simulink model "Magman_PID"  (R2016b)
settings: Solver=VariableStepAuto  StartTime=0.0  StopTime=60  RelTol=1e-3
values from neighbouring files (symbols this model uses):
  a = 5.713e-09    [LQI_script.m]    (also in PID_script.m = 4.367e-09; fminsim.m = block.InputPort(3).Data; model_generation.m = 4.367e-09)
  b = 0.000324    [LQI_script.m]    (also in PID_script.m = 0.0002827; fminsim.m = block.InputPort(4).Data; model_generation.m = 0.0002827)
  c = 0.0005    [PID_script.m]
  h = 0.01    [LQI_script.m]    (also in PID_script.m; model_generation.m)
  x1 = 0.02525    [LQI_script.m]    (also in PID_script.m; fminsim.m = block.InputPort(5).Data; model_generation.m)
  x2 = 0.05    [LQI_script.m]    (also in PID_script.m; fminsim.m = block.InputPort(6).Data; model_generation.m)
  x3 = 0.0751    [LQI_script.m]    (also in PID_script.m; fminsim.m = block.InputPort(7).Data; model_generation.m)
  x4 = 0.103    [LQI_script.m]    (also in PID_script.m; fminsim.m = block.InputPort(8).Data; model_generation.m)
undefined symbols (not defined in the file or in its folder): Ad, Bd, Cd, Dd, Humusoft, MF634
libraries: simulink x12, dspsrcs4 x1, sldrtlib x1
settings Model: Creator=Andres  LastModifiedBy=ajurisson

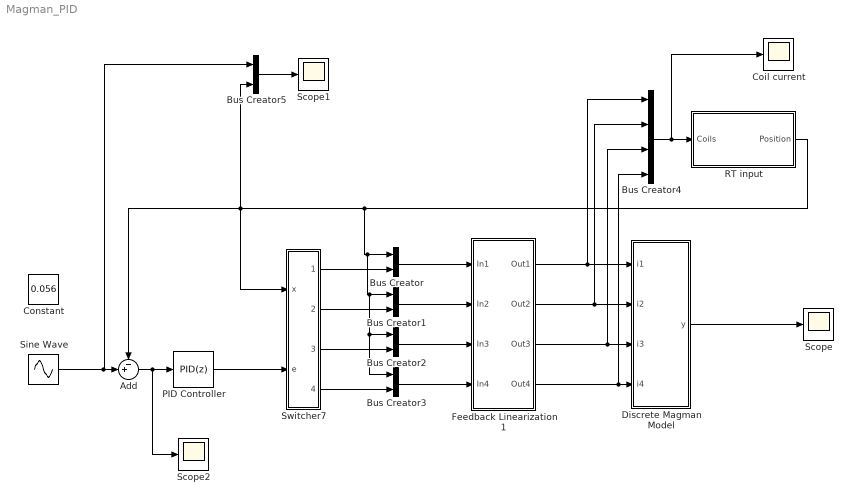
== system Magman_PID ==
  Add : Sum  Inputs=-+|
  Bus Creator{,1..3,5} (5 alike) : BusCreator  Inputs=2
  Bus Creator4 : BusCreator  Inputs=4
  Coil current : Scope
  Constant : Constant  Value=0.056
  Discrete Magman Model : Subsystem
  Feedback Linearization1 : Subsystem
  PID Controller : simulink/Continuous/PID Controller  Controller=PID  TimeDomain=Discrete-time  SampleTime=-1  IntegratorMethod=Trapezoidal  FilterMethod=Trapezoidal  Form=Parallel  UseFilter=on  ControllerParametersSource=internal  P=2.2  I=1  D=5  N=1000  InitialConditionSource=internal  InitialConditionForIntegrator=0  InitialConditionForFilter=0  ExternalReset=none  LimitOutput=off  UpperSaturationLimit=inf  LowerSaturationLimit=-inf  LinearizeAsGain=on  AntiWindupMode=none  Kb=1  TrackingMode=off  Kt=1  PParamMin=[]  PParamMax=[]  IParamMin=[]  IParamMax=[]  DParamMin=[]  DParamMax=[]  NParamMin=[]  NParamMax=[]  KbParamMin=[]  KbParamMax=[]  KtParamMin=[]  KtParamMax=[]  POutMin=[]  POutMax=[]  IOutMin=[]  IOutMax=[]  DOutMin=[]  DOutMax=[]  NOutMin=[]  NOutMax=[]  KbOutMin=[]  KbOutMax=[]  KtOutMin=[]  KtOutMax=[]  IntegratorOutMin=[]  IntegratorOutMax=[]  FilterOutMin=[]  FilterOutMax=[]  SumOutMin=[]  SumOutMax=[]  SumI1OutMin=[]  SumI1OutMax=[]  SumI2OutMin=[]  SumI2OutMax=[]  SumI3OutMin=[]  SumI3OutMax=[]  SumDOutMin=[]  SumDOutMax=[]  SaturationOutMin=[]  SaturationOutMax=[]  IntegratorContinuousStateAttributes=''  IntegratorStateMustResolveToSignalObject=off  IntegratorRTWStateStorageClass=Auto  FilterContinuousStateAttributes=''  FilterStateMustResolveToSignalObject=off  FilterRTWStateStorageClass=Auto  DifferentiatorICPrevScaledInput=0  DifferentiatorOutMin=[]  DifferentiatorOutMax=[]
  RT input : Subsystem  mask{h=0.01, Port=['COM4';'COM5']}
      mask prompts: h "Sample time [s]:"; Port "Serial ports:"
      mask Display: disp('Magman')
  Scope : Scope
  Scope1 : Scope
  Scope2 : Scope
  Sine Wave : Sin  Amplitude=0.032  Bias=0.063  Frequency=1.2  SampleTime=0
  Switcher7 : Subsystem
  wires:
  Add/1 -> Scope2/1, PID Controller/1
  PID Controller/1 -> Switcher7/2(e)
  Switcher7/2(v2) -> Bus Creator1/2
  Switcher7/4(v4) -> Bus Creator3/2
  Switcher7/3(v3) -> Bus Creator2/2
  Switcher7/1(v1) -> Bus Creator/2
  Bus Creator/1 -> Feedback Linearization1/1(In1)
  Bus Creator1/1 -> Feedback Linearization1/2(In2)
  Bus Creator2/1 -> Feedback Linearization1/3(In3)
  Bus Creator3/1 -> Feedback Linearization1/4(In4)
  Feedback Linearization1/1(Out1) -> Bus Creator4/1, Discrete Magman Model/1(i1)
  Feedback Linearization1/3(Out3) -> Bus Creator4/3, Discrete Magman Model/3(i3)
  Feedback Linearization1/4(Out4) -> Bus Creator4/4, Discrete Magman Model/4(i4)
  Bus Creator5/1 -> Scope1/1
  Sine Wave/1 -> Bus Creator5/1, Add/2
  Feedback Linearization1/2(Out2) -> Bus Creator4/2, Discrete Magman Model/2(i2)
  Discrete Magman Model/1(y) -> Scope/1
  Bus Creator4/1 -> Coil current/1, RT input/1(Coils)
  RT input/1(Position) -> Bus Creator3/1, Bus Creator2/1, Bus Creator1/1, Bus Creator/1, Switcher7/1(x), Bus Creator5/2, Add/1

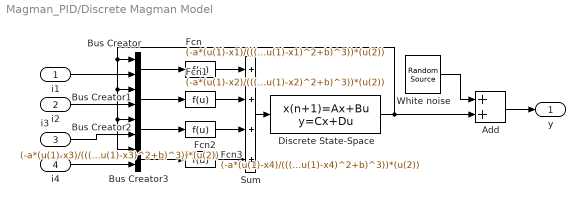
== system Magman_PID/Discrete Magman Model ==
  i1 : Inport
  i2 : Inport  Port=2
  i3 : Inport  Port=3
  i4 : Inport  Port=4
  Add : Sum
  Bus Creator{,1..3} (4 alike) : BusCreator  Inputs=2
  Discrete State-Space : DiscreteStateSpace  A=Ad  B=Bd  C=Cd  D=Dd  SampleTime=h
  Fcn : Fcn  Expr=(-a*(u(1)-x1)/(((u(1)-x1)^2+b)^3))*(u(2))
  Fcn1 : Fcn  Expr=(-a*(u(1)-x2)/(((u(1)-x2)^2+b)^3))*(u(2))
  Fcn2 : Fcn  Expr=(-a*(u(1)-x3)/(((u(1)-x3)^2+b)^3))*(u(2))
  Fcn3 : Fcn  Expr=(-a*(u(1)-x4)/(((u(1)-x4)^2+b)^3))*(u(2))
  Sum : Sum  Inputs=++++
  White noise : dspsrcs4/Random Source  SrcType=Gaussian  NormMethod=Ziggurat  CltLength=12  MinVal=0  MaxVal=1  MeanVal=0  VarVal=pos_var  RepMode=Not repeatable  rawSeed=1  IsInherit=off  SampMode=Discrete  SampTime=h  SampFrame=1  DataType=Double  OutComplex=Real  OutputFrames=off
  y : Outport
  wires:
  Fcn1/1 -> Sum/2
  Add/1 -> y/1
  Bus Creator3/1 -> Fcn3/1
  Bus Creator1/1 -> Fcn1/1
  i1/1 -> Bus Creator/2
  i2/1 -> Bus Creator1/2
  i3/1 -> Bus Creator2/2
  i4/1 -> Bus Creator3/2
  Sum/1 -> Discrete State-Space/1
  Fcn2/1 -> Sum/3
  Bus Creator2/1 -> Fcn2/1
  Fcn/1 -> Sum/1
  Fcn3/1 -> Sum/4
  Bus Creator/1 -> Fcn/1
  Discrete State-Space/1 -> Add/2, Bus Creator3/1, Bus Creator2/1, Bus Creator1/1, Bus Creator/1
  White noise/1 -> Add/1

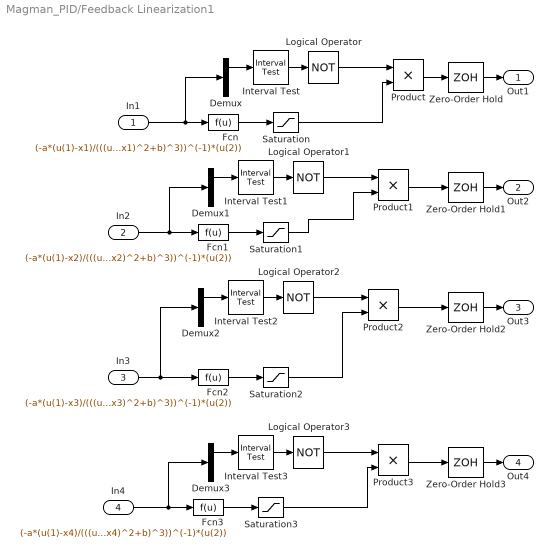
== system Magman_PID/Feedback Linearization1 ==
  In1 : Inport
  In2 : Inport  Port=2
  In3 : Inport  Port=3
  In4 : Inport  Port=4
  Demux{,1..3} (4 alike) : Demux  Outputs=2
  Fcn : Fcn  Expr=(-a*(u(1)-x1)/(((u(1)-x1)^2+b)^3))^(-1)*(u(2))
  Fcn1 : Fcn  Expr=(-a*(u(1)-x2)/(((u(1)-x2)^2+b)^3))^(-1)*(u(2))
  Fcn2 : Fcn  Expr=(-a*(u(1)-x3)/(((u(1)-x3)^2+b)^3))^(-1)*(u(2))
  Fcn3 : Fcn  Expr=(-a*(u(1)-x4)/(((u(1)-x4)^2+b)^3))^(-1)*(u(2))
  Interval Test : simulink/Logic and Bit Operations/Interval Test  IntervalClosedRight=on  uplimit=x1+c  IntervalClosedLeft=on  lowlimit=x1-c  OutDataTypeStr=boolean
  Interval Test1 : simulink/Logic and Bit Operations/Interval Test  IntervalClosedRight=on  uplimit=x2+c  IntervalClosedLeft=on  lowlimit=x2-c  OutDataTypeStr=boolean
  Interval Test2 : simulink/Logic and Bit Operations/Interval Test  IntervalClosedRight=on  uplimit=x3+c  IntervalClosedLeft=on  lowlimit=x3-c  OutDataTypeStr=boolean
  Interval Test3 : simulink/Logic and Bit Operations/Interval Test  IntervalClosedRight=on  uplimit=x4+c  IntervalClosedLeft=on  lowlimit=x4-c  OutDataTypeStr=boolean
  Logical Operator{,1..3} (4 alike) : Logic  Operator=NOT  AllPortsSameDT=off  OutDataTypeStr=boolean
  Product{,1..3} (4 alike) : Product
  Saturation{,1..3} (4 alike) : Saturate  UpperLimit=0.45  LowerLimit=0
  Zero-Order Hold{,1..3} (4 alike) : ZeroOrderHold  SampleTime=-1
  Out1 : Outport
  Out2 : Outport  Port=2
  Out3 : Outport  Port=3
  Out4 : Outport  Port=4
  wires:
  In1/1 -> Demux/1, Fcn/1
  Fcn3/1 -> Saturation3/1
  Fcn2/1 -> Saturation2/1
  Fcn1/1 -> Saturation1/1
  Fcn/1 -> Saturation/1
  Saturation/1 -> Product/2
  Demux/1 -> Interval Test/1
  Interval Test/1 -> Logical Operator/1
  Logical Operator/1 -> Product/1
  Product/1 -> Zero-Order Hold/1
  In2/1 -> Demux1/1, Fcn1/1
  Saturation1/1 -> Product1/2
  Demux1/1 -> Interval Test1/1
  Interval Test1/1 -> Logical Operator1/1
  Logical Operator1/1 -> Product1/1
  Product1/1 -> Zero-Order Hold1/1
  In3/1 -> Demux2/1, Fcn2/1
  Saturation2/1 -> Product2/2
  Demux2/1 -> Interval Test2/1
  Interval Test2/1 -> Logical Operator2/1
  Logical Operator2/1 -> Product2/1
  Product2/1 -> Zero-Order Hold2/1
  In4/1 -> Demux3/1, Fcn3/1
  Saturation3/1 -> Product3/2
  Demux3/1 -> Interval Test3/1
  Interval Test3/1 -> Logical Operator3/1
  Logical Operator3/1 -> Product3/1
  Product3/1 -> Zero-Order Hold3/1
  Zero-Order Hold/1 -> Out1/1
  Zero-Order Hold1/1 -> Out2/1
  Zero-Order Hold2/1 -> Out3/1
  Zero-Order Hold3/1 -> Out4/1

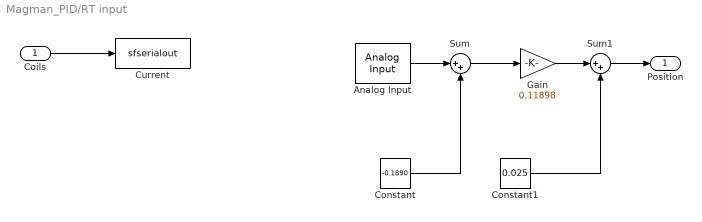
== system Magman_PID/RT input ==
  Coils : Inport
  Analog Input : sldrtlib/Analog Input  SampleTime=h  MaxMissedTicks=100  ShowMissedTicks=off  YieldWhenWaiting=off  DrvName=Humusoft/MF634  DrvAddress=4294967295  DrvOptions=0  Channels=1  RangeMode=2  VoltRange=1  DataType=1
      settings: AttributesFormatString=Humusoft\nMF634 [auto]
  Constant : Constant  Value=-0.1890
  Constant1 : Constant  Value=0.025
  Current : S-Function  FunctionName=sfserialout  Parameters=h, com  SFunctionDeploymentMode=off  EnableBusSupport=off  mask(Serial Out){h=h, Port=Port}
      mask prompts: h "Sample time:"; Port "Serial port:"
      mask help: Serial line output block
      mask init:
      | com(1)              = rs232('GetParams','default'); % get default RS232 parameters
      | com(1).Port         = Port(1,:);                    % define port number
      | com(1).BaudRate     = 115200;                       % define Baud rate
      | com(1).ReadTimeout  = 1;                            % define short timeout
      | com(1).WriteTimeout = 1;                            % define short timeout
      | rs232('open',com(1));                               % open the port
      | 
      | com(2)              = rs232('GetParams','default'); % get default RS232 parameters
      | com(2).Port         = Port(2,:);                    % define port number
      | com(2).BaudRate     = 115200;                       % define Baud rate
      | com(2).ReadTimeout  = 1;                            % define short timeout
      | com(2).WriteTimeout = 1;                            % define short timeout
      | rs232('open',com(2)); 
      | 
      | %com(1) = serial(['COM' num2str(Port(1))],'BaudRate',115200,'Timeout',1,'DataBits',8,'StopBits',1,'Parity','none','Terminator','CR/LF');
      | %com(2) = serial(['COM' num2str(Port(2))],'BaudRate',115200,'Timeout',1,'DataBits',8,'StopBits',1,'Parity','none','Terminator','CR/LF');
      | %fopen(com);
      mask Help: Serial Out block is designed as a serial communication output block for real time data acquisition, signal processing and control applications.
      mask Display: disp('Coils');
  Gain : Gain  Gain=0.11898
  Sum : Sum  Inputs=|++
  Sum1 : Sum  Inputs=|++
  Position : Outport
  wires:
  Coils/1 -> Current/1
  Analog Input/1 -> Sum/1
  Constant/1 -> Sum/2
  Sum/1 -> Gain/1
  Gain/1 -> Sum1/1
  Sum1/1 -> Position/1
  Constant1/1 -> Sum1/2

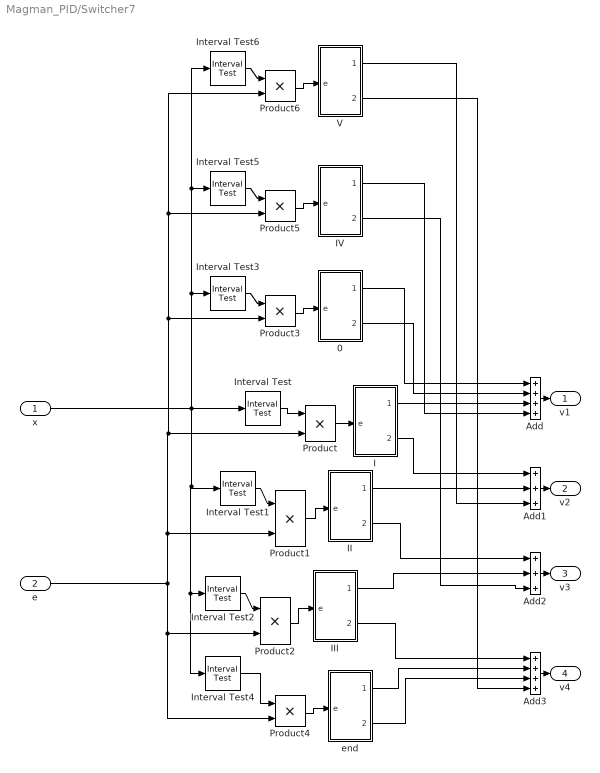
== system Magman_PID/Switcher7 ==
  x : Inport
  e : Inport  Port=2
  0 : Subsystem
  Add : Sum  Inputs=++++
  Add1 : Sum  Inputs=+++
  Add2 : Sum  Inputs=+++
  Add3 : Sum  Inputs=++++
  I : Subsystem
  II : Subsystem
  III : Subsystem
  IV : Subsystem
  Interval Test : simulink/Logic and Bit Operations/Interval Test  IntervalClosedRight=off  uplimit=x2-c  IntervalClosedLeft=on  lowlimit=x1-c  OutDataTypeStr=boolean
  Interval Test1 : simulink/Logic and Bit Operations/Interval Test  IntervalClosedRight=off  uplimit=x3-c  IntervalClosedLeft=off  lowlimit=x2+c  OutDataTypeStr=boolean
  Interval Test2 : simulink/Logic and Bit Operations/Interval Test  IntervalClosedRight=on  uplimit=x4+c  IntervalClosedLeft=off  lowlimit=x3+c  OutDataTypeStr=boolean
  Interval Test3 : simulink/Logic and Bit Operations/Interval Test  IntervalClosedRight=off  uplimit=x1-c  IntervalClosedLeft=on  lowlimit=0  OutDataTypeStr=boolean
  Interval Test4 : simulink/Logic and Bit Operations/Interval Test  IntervalClosedRight=on  uplimit=inf  IntervalClosedLeft=off  lowlimit=x4+c  OutDataTypeStr=boolean
  Interval Test5 : simulink/Logic and Bit Operations/Interval Test  IntervalClosedRight=on  uplimit=x2+c  IntervalClosedLeft=on  lowlimit=x2-c  OutDataTypeStr=boolean
  Interval Test6 : simulink/Logic and Bit Operations/Interval Test  IntervalClosedRight=on  uplimit=x3+c  IntervalClosedLeft=on  lowlimit=x3-c  OutDataTypeStr=boolean
  Product{,1..6} (7 alike) : Product
  V : Subsystem
  end : Subsystem
  v1 : Outport
  v2 : Outport  Port=2
  v3 : Outport  Port=3
  v4 : Outport  Port=4
  wires:
  Interval Test/1 -> Product/1
  Product/1 -> I/1(e)
  Add/1 -> v1/1
  Add1/1 -> v2/1
  Add2/1 -> v3/1
  Add3/1 -> v4/1
  I/2(Right coil) -> Add1/1
  Interval Test1/1 -> Product1/1
  Product1/1 -> II/1(e)
  II/1(Left coil) -> Add1/2
  II/2(Right coil) -> Add2/1
  Interval Test2/1 -> Product2/1
  Product2/1 -> III/1(e)
  III/1(Left coil) -> Add2/2
  III/2(Right coil) -> Add3/1
  Interval Test3/1 -> Product3/1
  Product3/1 -> 0/1(e)
  0/1(Left coil) -> Add/1
  I/1(Left coil) -> Add/3
  0/2(Right coil) -> Add/2
  Interval Test4/1 -> Product4/1
  Product4/1 -> end/1(e)
  end/1(Left coil) -> Add3/2
  end/2(Right coil) -> Add3/3
  Interval Test5/1 -> Product5/1
  Product5/1 -> IV/1(e)
  IV/1(Left coil) -> Add/4
  IV/2(Right coil) -> Add2/3
  Interval Test6/1 -> Product6/1
  Product6/1 -> V/1(e)
  V/1(Left coil) -> Add1/3
  V/2(Right coil) -> Add3/4
  x/1 -> Interval Test6/1, Interval Test5/1, Interval Test3/1, Interval Test4/1, Interval Test2/1, Interval Test1/1, Interval Test/1
  e/1 -> Product6/2, Product5/2, Product3/2, Product/2, Product1/2, Product4/2, Product2/2

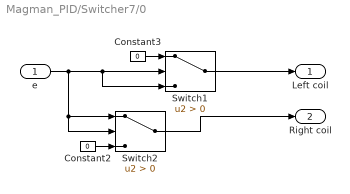
== system Magman_PID/Switcher7/0 ==
  e : Inport
  Constant2 : Constant  Value=0
  Constant3 : Constant  Value=0
  Switch1 : Switch  Criteria=u2 > Threshold
  Switch2 : Switch  Criteria=u2 > Threshold
  Left coil : Outport
  Right coil : Outport  Port=2
  wires:
  Switch1/1 -> Left coil/1
  Constant3/1 -> Switch1/1
  e/1 -> Switch2/1, Switch2/2, Switch1/3, Switch1/2
  Switch2/1 -> Right coil/1
  Constant2/1 -> Switch2/3

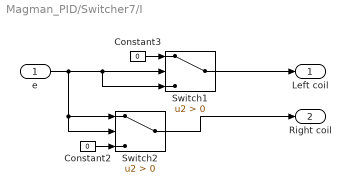
== system Magman_PID/Switcher7/I ==
  e : Inport
  Constant2 : Constant  Value=0
  Constant3 : Constant  Value=0
  Switch1 : Switch  Criteria=u2 > Threshold
  Switch2 : Switch  Criteria=u2 > Threshold
  Left coil : Outport
  Right coil : Outport  Port=2
  wires:
  Switch1/1 -> Left coil/1
  Constant3/1 -> Switch1/1
  e/1 -> Switch2/1, Switch2/2, Switch1/3, Switch1/2
  Switch2/1 -> Right coil/1
  Constant2/1 -> Switch2/3

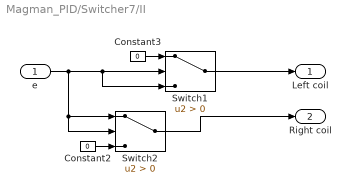
== system Magman_PID/Switcher7/II ==
  e : Inport
  Constant2 : Constant  Value=0
  Constant3 : Constant  Value=0
  Switch1 : Switch  Criteria=u2 > Threshold
  Switch2 : Switch  Criteria=u2 > Threshold
  Left coil : Outport
  Right coil : Outport  Port=2
  wires:
  Switch1/1 -> Left coil/1
  Constant3/1 -> Switch1/1
  e/1 -> Switch2/1, Switch2/2, Switch1/3, Switch1/2
  Switch2/1 -> Right coil/1
  Constant2/1 -> Switch2/3

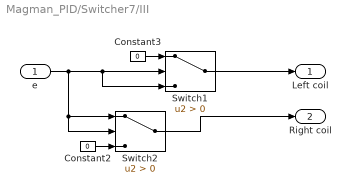
== system Magman_PID/Switcher7/III ==
  e : Inport
  Constant2 : Constant  Value=0
  Constant3 : Constant  Value=0
  Switch1 : Switch  Criteria=u2 > Threshold
  Switch2 : Switch  Criteria=u2 > Threshold
  Left coil : Outport
  Right coil : Outport  Port=2
  wires:
  Switch1/1 -> Left coil/1
  Constant3/1 -> Switch1/1
  e/1 -> Switch2/1, Switch2/2, Switch1/3, Switch1/2
  Switch2/1 -> Right coil/1
  Constant2/1 -> Switch2/3

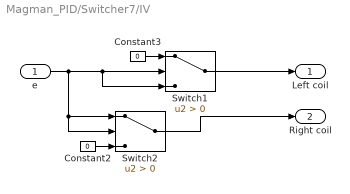
== system Magman_PID/Switcher7/IV ==
  e : Inport
  Constant2 : Constant  Value=0
  Constant3 : Constant  Value=0
  Switch1 : Switch  Criteria=u2 > Threshold
  Switch2 : Switch  Criteria=u2 > Threshold
  Left coil : Outport
  Right coil : Outport  Port=2
  wires:
  Switch1/1 -> Left coil/1
  Constant3/1 -> Switch1/1
  e/1 -> Switch2/1, Switch2/2, Switch1/3, Switch1/2
  Switch2/1 -> Right coil/1
  Constant2/1 -> Switch2/3

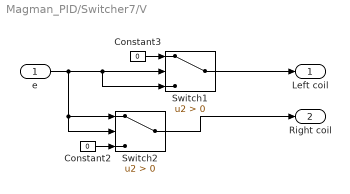
== system Magman_PID/Switcher7/V ==
  e : Inport
  Constant2 : Constant  Value=0
  Constant3 : Constant  Value=0
  Switch1 : Switch  Criteria=u2 > Threshold
  Switch2 : Switch  Criteria=u2 > Threshold
  Left coil : Outport
  Right coil : Outport  Port=2
  wires:
  Switch1/1 -> Left coil/1
  Constant3/1 -> Switch1/1
  e/1 -> Switch2/1, Switch2/2, Switch1/3, Switch1/2
  Switch2/1 -> Right coil/1
  Constant2/1 -> Switch2/3

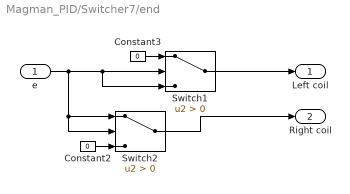
== system Magman_PID/Switcher7/end ==
  e : Inport
  Constant2 : Constant  Value=0
  Constant3 : Constant  Value=0
  Switch1 : Switch  Criteria=u2 > Threshold
  Switch2 : Switch  Criteria=u2 > Threshold
  Left coil : Outport
  Right coil : Outport  Port=2
  wires:
  Switch1/1 -> Left coil/1
  Constant3/1 -> Switch1/1
  e/1 -> Switch2/1, Switch2/2, Switch1/3, Switch1/2
  Switch2/1 -> Right coil/1
  Constant2/1 -> Switch2/3
